simulink model "sampleModel2012"  (R2023a)
settings: Solver=VariableStepAuto  StartTime=0.0  StopTime=10.0  RelTol=1e-3
libraries: hdlsllib x9, simulink x1
settings Model: Creator=user1  LastModifiedBy=user1

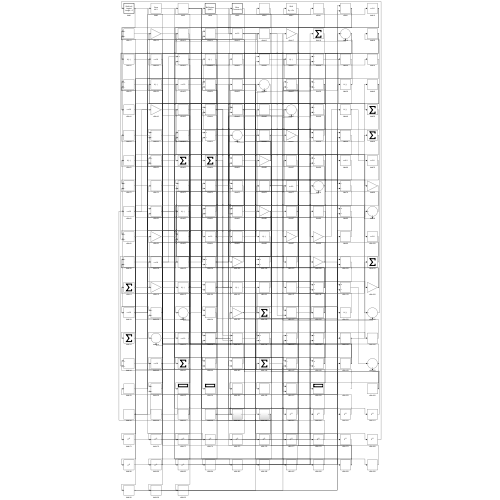
[thumbnail: Simulink's stored preview of the top-level diagram]
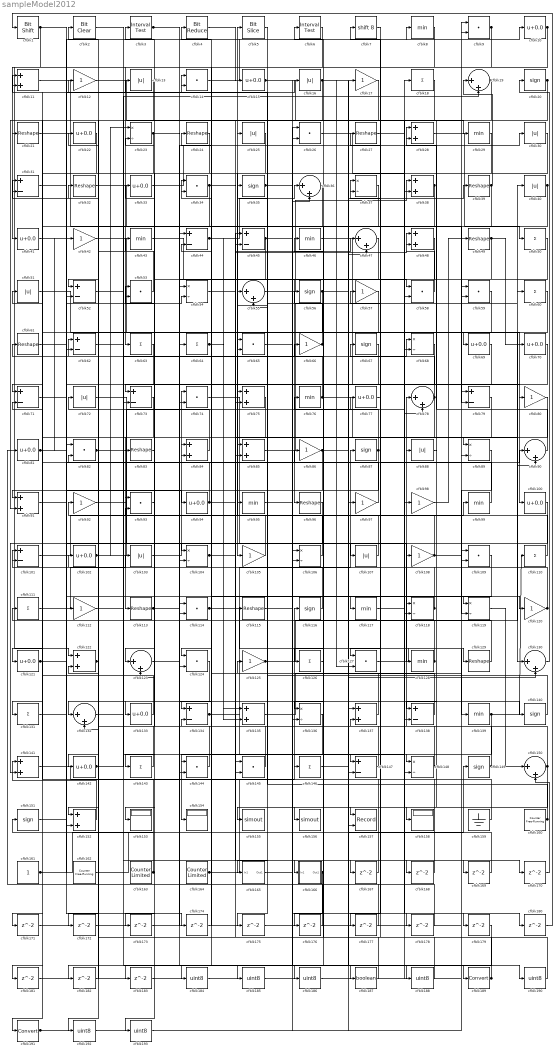
== system sampleModel2012 ==
  cfblk1 : hdlsllib/Logic and Bit Operations/Bit Shift  mode=Shift Left Logical  N=0
  cfblk{10,15,22,33,41,69..70,77,81,94,100,102,121,133,142} (15 alike) : Bias  Bias=0.0  SaturateOnIntegerOverflow=off
  cfblk{31,44..45,52,62,71,73,79,101,134,138,147} (12 alike) : Sum  Inputs=+-
  cfblk{13,16,25,30,40,51,72,88,103,107} (10 alike) : Abs  SaturateOnIntegerOverflow=off
  cfblk{23,37,54,68,89,104,106,118..119,136,148} (11 alike) : Product  Inputs=*/  RndMeth=Zero  SaturateOnIntegerOverflow=on
  cfblk{12,17,42,57,66,80,86,92,97..98,105,108,112,120,125} (15 alike) : Gain
  cfblk{9,14,26,34,53,58..59,65,74,82,93,109,114,124,127,144..145} (17 alike) : DotProduct  OutDataTypeStr=Inherit: Inherit via internal rule
  cfblk{11,28,38,48,75,84..85,91,122,135,137,141,152} (13 alike) : Sum
  cfblk{18,50,60,63..64,110..111,126,131,143,146} (11 alike) : Sum  Inputs=+
  cfblk{21,24,27,32,39,49,61,83,96,113,115,129} (12 alike) : Reshape
  cfblk{20,35,56,67,87,116,140,149,151} (9 alike) : Signum
  cfblk{8,29,43,46,76,95,99,117,128,139} (10 alike) : MinMax
  cfblk{19,36,47,55,78,90,123,130,132,150} (10 alike) : Sum  Inputs=|++
  cfblk153 : Display
  cfblk154 : Display
  cfblk155 : ToWorkspace  VariableName=simout  SaveFormat=Timeseries  SampleTime=-1
  cfblk156 : ToWorkspace  VariableName=simout  SaveFormat=Timeseries  SampleTime=-1
  cfblk157 : Record  FileSettingsInternal="{\"entries\":[{\"content\":{\"excelSettings\":{\"content\":{},\"type\":\"Streamout.ExcelSettings\"}},\"type\":\"Streamout.FileSettingStorage\",\"uuid\":\"\"}],\"packageUris\":[\"http:\\/\\/schema.mathworks.com\\/mf0\\/streamout_blocks\\/R2020a\"],\"version\":\"1.0\"}"  Layout=[1 1]  SignalsInternal="{\"entries\":[{\"content\":{\"signals\":[{\"content\":{\"blockPath\":[],\"dimensions\":[1],\"domain\":\"\",\"lineColor\":\"#a2142f\",\"plots\":[1],\"port\":1,\"signalID\":5926,\"signalName\":\"XY Graph:1\"},\"type\":\"RecordBlkView.Signal\",\"uuid\":\"\"},{\"content\":{\"blockPath\":[],\"dimensions\":[1],\"domain\":\"\",\"lineColor\":\"#139fff\",\"plots\":[1],\"port\":2,\"signalID\":5929,\"signalName\":\"XY Graph:2\"},\"type\":\"RecordBlkView.Signal\",\"uuid\":\"\"}]},\"type\":\"RecordBlkView.InputSignals\",\"uuid\":\"\"}],\"packageUris\":[\"http:\\/\\/schema.mathworks.com\\/mf0\\/streamout_blocks\\/R2020a\"],\"version\":\"1.0\"}"  VisualizationBindings="{\"xyplotplugin\":{\"info\":[{\"series\":[{\"bindingParametersList\":[{\"parameter\":\"X-Axis\",\"signalID\":5926,\"signalName\":\"XY Graph:1\"},{\"parameter\":\"Y-Axis\",\"signalID\":5929,\"signalName\":\"XY Graph:2\"}],\"seriesID\":65058}],\"subplotID\":1}]}}"  CompatibilityTag=XY  st=-1
  cfblk158 : Display
  cfblk159 : Ground
  cfblk160 : hdlsllib/Sources/Counter Free-Running  NumBits=16  tsamp=-1
  cfblk161 : Constant  SampleTime=-1
  cfblk162 : hdlsllib/Sources/Counter Free-Running  NumBits=16  tsamp=-1
  cfblk163 : hdlsllib/Sources/Counter Limited  uplimit=7  tsamp=-1
  cfblk164 : hdlsllib/Sources/Counter Limited  uplimit=7  tsamp=-1
  cfblk165 : Subsystem
      settings: LibrarySourceBlock=|
      | hdlsllib/Ports &
      | Subsystems/Subsystem
  cfblk166 : Subsystem
      settings: LibrarySourceBlock=|
      | hdlsllib/Ports &
      | Subsystems/Subsystem
  cfblk{167..183} (17 alike) : Delay  SampleTime=1
  cfblk{184..186,188,190,192..193} (7 alike) : DataTypeConversion  OutDataTypeStr=uint8  SaturateOnIntegerOverflow=off  RndMeth=Floor
  cfblk187 : DataTypeConversion  OutDataTypeStr=boolean  SaturateOnIntegerOverflow=off  RndMeth=Floor
  cfblk189 : DataTypeConversion  SaturateOnIntegerOverflow=off  RndMeth=Floor
  cfblk191 : DataTypeConversion  SaturateOnIntegerOverflow=off  RndMeth=Floor
  cfblk2 : simulink/Logic and Bit Operations/Bit Clear  iBit=0
      settings: LibrarySourceBlock=|
      | hdlsllib/Logic and Bit
      | Operations/Bit Clear
  cfblk3 : hdlsllib/Logic and Bit Operations/Interval Test  IntervalClosedRight=on  uplimit=0.5  IntervalClosedLeft=on  lowlimit=-0.5  OutDataTypeStr=boolean
  cfblk4 : hdlsllib/Logic and Bit Operations/Bit Reduce  mode=AND
  cfblk5 : hdlsllib/Logic and Bit Operations/Bit Slice  lidx=7  ridx=0
  cfblk6 : hdlsllib/Logic and Bit Operations/Interval Test  IntervalClosedRight=on  uplimit=0.5  IntervalClosedLeft=on  lowlimit=-0.5  OutDataTypeStr=boolean
  cfblk7 : ArithShift  BitShiftNumber=8
  wires:
  cfblk81/1 -> cfblk42/1, cfblk93/1
  cfblk10/1 -> cfblk63/1, cfblk127/1
  cfblk106/1 -> cfblk5/1
  cfblk1/1 -> cfblk122/1, cfblk118/1
  cfblk73/1 -> cfblk113/1
  cfblk134/1 -> cfblk87/1, cfblk157/2, cfblk4/1
  cfblk98/1 -> cfblk49/1
  cfblk3/1 -> cfblk140/1, cfblk167/1, cfblk185/1
  cfblk82/1 -> cfblk144/2, cfblk187/1
  cfblk83/1 -> cfblk133/1
  cfblk11/1 -> cfblk79/1
  cfblk119/1 -> cfblk150/1
  cfblk14/1 -> cfblk8/1
  cfblk142/1 -> cfblk19/2, cfblk172/1
  cfblk28/1 -> cfblk50/1
  cfblk49/1 -> cfblk96/1, cfblk70/1
  cfblk141/1 -> cfblk116/1
  cfblk42/1 -> cfblk100/1
  cfblk63/1 -> cfblk73/1
  cfblk55/1 -> cfblk38/1
  cfblk94/1 -> cfblk11/1, cfblk170/1
  cfblk46/1 -> cfblk79/2
  cfblk30/1 -> cfblk105/1
  cfblk99/1 -> cfblk57/1
  cfblk67/1 -> cfblk153/1
  cfblk62/1 -> cfblk147/1
  cfblk146/1 -> cfblk189/1
  cfblk124/1 -> cfblk132/1
  cfblk163/1 -> cfblk151/1, cfblk32/1
  cfblk115/1 -> cfblk90/1
  cfblk36/1 -> cfblk52/1
  cfblk149/1 -> cfblk78/1, cfblk53/2, cfblk23/2
  cfblk102/1 -> cfblk30/1, cfblk23/1
  cfblk58/1 -> cfblk48/1
  cfblk120/1 -> cfblk56/1, cfblk13/1
  cfblk110/1 -> cfblk92/1
  cfblk4/1 -> cfblk15/1
  cfblk84/1 -> cfblk72/1
  cfblk44/1 -> cfblk36/1, cfblk115/1, cfblk135/2
  cfblk126/1 -> cfblk6/1
  cfblk85/1 -> cfblk40/1
  cfblk59/1 -> cfblk191/1
  cfblk143/1 -> cfblk61/1
  cfblk60/1 -> cfblk157/1
  cfblk57/1 -> cfblk156/1
  cfblk86/1 -> cfblk39/1, cfblk181/1, cfblk182/1
  cfblk35/1 -> cfblk148/2, cfblk190/1
  cfblk164/1 -> cfblk26/1, cfblk89/2
  cfblk152/1 -> cfblk141/1
  cfblk93/1 -> cfblk43/1
  cfblk127/1 -> cfblk129/1
  cfblk122/1 -> cfblk62/1, cfblk102/1
  cfblk37/1 -> cfblk143/1
  cfblk25/1 -> cfblk71/1
  cfblk125/1 -> cfblk60/1, cfblk55/2
  cfblk27/1 -> cfblk98/1
  cfblk88/1 -> cfblk158/1
  cfblk9/1 -> cfblk41/1, cfblk74/2
  cfblk111/1 -> cfblk103/1
  cfblk103/1 -> cfblk74/1
  cfblk90/1 -> cfblk28/1
  cfblk132/1 -> cfblk68/1
  cfblk32/1 -> cfblk78/2
  cfblk116/1 -> cfblk3/1
  cfblk29/1 -> cfblk142/1
  cfblk144/1 -> cfblk53/1
  cfblk40/1 -> cfblk126/1, cfblk95/1
  cfblk39/1 -> cfblk121/1, cfblk19/1
  cfblk43/1 -> cfblk75/1
  cfblk133/1 -> cfblk111/1
  cfblk136/1 -> cfblk154/1
  cfblk19/1 -> cfblk138/1, cfblk132/2
  cfblk96/1 -> cfblk141/2
  cfblk18/1 -> cfblk21/1
  cfblk15/1 -> cfblk97/1, cfblk118/2, cfblk58/1
  cfblk150/1 -> cfblk155/1, cfblk33/1
  cfblk118/1 -> cfblk37/1, cfblk82/2, cfblk34/2
  cfblk20/1 -> cfblk148/1, cfblk85/2
  cfblk147/1 -> cfblk66/1
  cfblk140/1 -> cfblk35/1
  cfblk101/1 -> cfblk36/2
  cfblk76/1 -> cfblk90/2, cfblk31/2, cfblk130/2
  cfblk48/1 -> cfblk124/1
  cfblk104/1 -> cfblk48/2, cfblk99/1
  cfblk148/1 -> cfblk12/1, cfblk31/1
  cfblk23/1 -> cfblk62/2, cfblk58/2
  cfblk78/1 -> cfblk123/1, cfblk27/1
  cfblk135/1 -> cfblk9/2
  cfblk80/1 -> cfblk114/2
  cfblk72/1 -> cfblk124/2
  cfblk21/1 -> cfblk64/1
  cfblk71/1 -> cfblk107/1
  cfblk95/1 -> cfblk77/1
  cfblk100/1 -> cfblk106/2
  cfblk7/1 -> cfblk117/1
  cfblk56/1 -> cfblk152/1, cfblk47/2
  cfblk66/1 -> cfblk14/1, cfblk11/2
  cfblk131/1 -> cfblk84/1
  cfblk160/1 -> cfblk125/1, cfblk76/1
  cfblk137/1 -> cfblk44/2
  cfblk61/1 -> cfblk94/1
  cfblk139/1 -> cfblk110/1, cfblk165/1(In1)
  cfblk6/1 -> cfblk73/2
  cfblk26/1 -> cfblk38/2
  cfblk17/1 -> cfblk65/1
  cfblk151/1 -> cfblk10/1
  cfblk53/1 -> cfblk22/1
  cfblk105/1 -> cfblk84/2
  cfblk70/1 -> cfblk145/2
  cfblk138/1 -> cfblk55/1
  cfblk128/1 -> cfblk37/2, cfblk51/1
  cfblk33/1 -> cfblk25/1
  cfblk166/1(Out1) -> cfblk81/1, cfblk176/1
  cfblk161/1 -> cfblk112/1, cfblk149/1
  cfblk107/1 -> cfblk86/1
  cfblk74/1 -> cfblk128/1
  cfblk79/1 -> cfblk91/1
  cfblk69/1 -> cfblk123/2
  cfblk121/1 -> cfblk54/2, cfblk16/1
  cfblk91/1 -> cfblk82/1
  cfblk97/1 -> cfblk34/1
  cfblk87/1 -> cfblk46/1, cfblk193/1
  cfblk47/1 -> cfblk85/1
  cfblk65/1 -> cfblk119/1
  cfblk108/1 -> cfblk120/1, cfblk7/1
  cfblk129/1 -> cfblk101/1
  cfblk68/1 -> cfblk136/1
  cfblk13/1 -> cfblk131/1
  cfblk145/1 -> cfblk101/2
  cfblk123/1 -> cfblk28/2
  cfblk130/1 -> cfblk20/1
  cfblk54/1 -> cfblk108/1
  cfblk38/1 -> cfblk75/2, cfblk104/2
  cfblk64/1 -> cfblk24/1, cfblk104/1, cfblk135/1
  cfblk159/1 -> cfblk65/2
  cfblk113/1 -> cfblk88/1, cfblk166/1(In1), cfblk93/2
  cfblk45/1 -> cfblk83/1, cfblk69/1, cfblk169/1
  cfblk89/1 -> cfblk119/2
  cfblk34/1 -> cfblk152/2, cfblk89/1, cfblk52/2
  cfblk112/1 -> cfblk144/1
  cfblk162/1 -> cfblk136/2
  cfblk41/1 -> cfblk80/1
  cfblk114/1 -> cfblk139/1, cfblk47/1
  cfblk16/1 -> cfblk91/2, cfblk127/2, cfblk180/1
  cfblk51/1 -> cfblk130/1
  cfblk92/1 -> cfblk45/2
  cfblk8/1 -> cfblk134/1
  cfblk12/1 -> cfblk29/1
  cfblk167/1 -> cfblk71/2
  cfblk52/1 -> cfblk168/1
  cfblk168/1 -> cfblk54/1
  cfblk169/1 -> cfblk137/1
  cfblk170/1 -> cfblk150/2
  cfblk22/1 -> cfblk171/1
  cfblk171/1 -> cfblk9/1
  cfblk172/1 -> cfblk44/1
  cfblk75/1 -> cfblk173/1
  cfblk173/1 -> cfblk138/2
  cfblk31/1 -> cfblk174/1
  cfblk174/1 -> cfblk14/2
  cfblk5/1 -> cfblk175/1
  cfblk175/1 -> cfblk106/1
  cfblk176/1 -> cfblk134/2
  cfblk77/1 -> cfblk177/1
  cfblk177/1 -> cfblk45/1
  cfblk165/1(Out1) -> cfblk178/1
  cfblk178/1 -> cfblk114/1
  cfblk117/1 -> cfblk179/1
  cfblk180/1 -> cfblk1/1
  cfblk181/1 -> cfblk147/2
  cfblk182/1 -> cfblk122/2
  cfblk24/1 -> cfblk183/1
  cfblk183/1 -> cfblk18/1
  cfblk109/1 -> cfblk184/1
  cfblk184/1 -> cfblk68/2
  cfblk185/1 -> cfblk109/1
  cfblk50/1 -> cfblk186/1
  cfblk186/1 -> cfblk109/2
  cfblk187/1 -> cfblk2/1
  cfblk2/1 -> cfblk188/1
  cfblk188/1 -> cfblk67/1
  cfblk189/1 -> cfblk137/2, cfblk145/1
  cfblk190/1 -> cfblk146/1
  cfblk191/1 -> cfblk26/2, cfblk17/1
  cfblk179/1 -> cfblk192/1
  cfblk192/1 -> cfblk59/1
  cfblk193/1 -> cfblk59/2

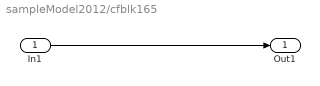
== system sampleModel2012/cfblk165 ==
  In1 : Inport
  Out1 : Outport
  wires:
  In1/1 -> Out1/1

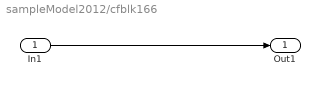
== system sampleModel2012/cfblk166 ==
  In1 : Inport
  Out1 : Outport
  wires:
  In1/1 -> Out1/1
